simulink model "cobem_IMC"  (R2018a)
settings: Solver=FixedStepAuto  StartTime=0.0  StopTime=tfinal  FixedStep=dt  RelTol=1e-3
values from neighbouring files (symbols this model uses):
  a1 = 0.0190125110732    [PSO_workspace_PID_v1.0_agoravai_refnova.mat]    (also in cobem_IMC_script.m; teste_linearizacao.m)
  a2 = 0.594107643424    [PSO_workspace_PID_v1.0_agoravai_refnova.mat]    (also in cobem_IMC_script.m = num2/den2; teste_linearizacao.m = num2/den2)
  a3 = 0.0893725569407    [PSO_workspace_PID_v1.0_agoravai_refnova.mat]    (also in cobem_IMC_script.m = num3/den3; teste_linearizacao.m = num3/den3)
  a4 = 0.0670294177055    [PSO_workspace_PID_v1.0_agoravai_refnova.mat]    (also in cobem_IMC_script.m = num4/den4; teste_linearizacao.m = num4/den4)
  h10 = 0.3    [PSO_workspace_PID_v1.0_agoravai_refnova.mat]    (also in cobem_IMC_script.m)
  H1max = 1    [PSO_workspace_PID_v1.0_agoravai_refnova.mat]    (also in cobem_IMC_script.m; teste_linearizacao.m)
  h20 = 0.1    [PSO_workspace_PID_v1.0_agoravai_refnova.mat]    (also in cobem_IMC_script.m)
  H2max = 1    [PSO_workspace_PID_v1.0_agoravai_refnova.mat]    (also in cobem_IMC_script.m; teste_linearizacao.m)
  KpIMC = (tau1+tau2)/(K*lambda)    [cobem_IMC_script.m]
  N = 100    [PSO_workspace_PID_v1.0_agoravai_refnova.mat]    (also in cobem_IMC_script.m)
  satF_inf = 10    [PSO_workspace_PID_v1.0_agoravai_refnova.mat]    (also in cobem_IMC_script.m)
  satF_sup = 90    [PSO_workspace_PID_v1.0_agoravai_refnova.mat]    (also in cobem_IMC_script.m)
  TdIMC = (tau1*tau2)/(tau1+tau2)    (= 1.32135382724)    [cobem_IMC_script.m]
  TiIMC = (tau1+tau2)    (= 6.506)    [cobem_IMC_script.m]
settings Model: Creator=generic-user  LastModifiedBy=generic-user

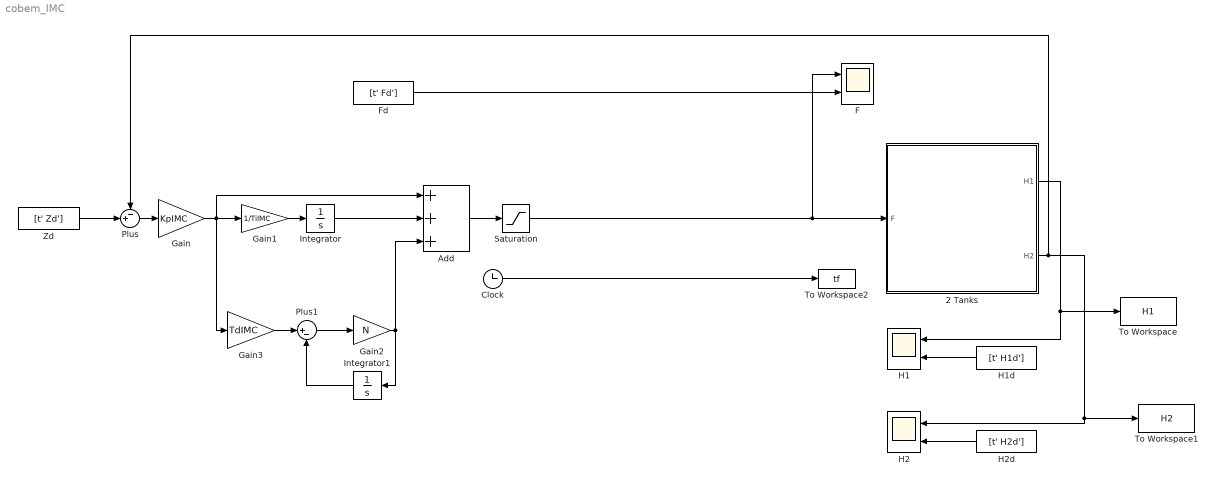
== system cobem_IMC ==
  2 Tanks : Subsystem
  Add : Sum  Inputs=3
  Clock : Clock
  F : Scope  NumInputPorts=2
  Fd : FromWorkspace  VariableName=[t' Fd']  SampleTime=0  OutputAfterFinalValue=Holding final value
  Gain : Gain  Gain=KpIMC
  Gain1 : Gain  Gain=1/TiIMC
  Gain2 : Gain  Gain=N
  Gain3 : Gain  Gain=TdIMC
  H1 : Scope  NumInputPorts=2
  H1d : FromWorkspace  VariableName=[t' H1d']  SampleTime=0  OutputAfterFinalValue=Holding final value
  H2 : Scope  NumInputPorts=2
  H2d : FromWorkspace  VariableName=[t' H2d']  SampleTime=0  OutputAfterFinalValue=Holding final value
  Integrator : Integrator
  Integrator1 : Integrator
  Plus : Sum  Inputs=-+|
  Plus1 : Sum  Inputs=|+-
  Saturation : Saturate  UpperLimit=satF_sup  LowerLimit=satF_inf
  To Workspace : ToWorkspace  VariableName=H1  SampleTime=-1
  To Workspace1 : ToWorkspace  VariableName=H2  SampleTime=-1
  To Workspace2 : ToWorkspace  VariableName=tf  SampleTime=-1
  Zd : FromWorkspace  VariableName=[t' Zd']  SampleTime=0  OutputAfterFinalValue=Holding final value
  wires:
  Zd/1 -> Plus/2
  H2d/1 -> H2/2
  2 Tanks/1(H1) -> To Workspace/1, H1/1
  Plus/1 -> Gain/1
  Fd/1 -> F/2
  Clock/1 -> To Workspace2/1
  2 Tanks/2(H2) -> To Workspace1/1, H2/1, Plus/1
  H1d/1 -> H1/2
  Add/1 -> Saturation/1
  Integrator/1 -> Add/2
  Gain/1 -> Gain3/1, Add/1, Gain1/1
  Gain1/1 -> Integrator/1
  Integrator1/1 -> Plus1/2
  Plus1/1 -> Gain2/1
  Gain2/1 -> Integrator1/1, Add/3
  Gain3/1 -> Plus1/1
  Saturation/1 -> F/1, 2 Tanks/1(F)

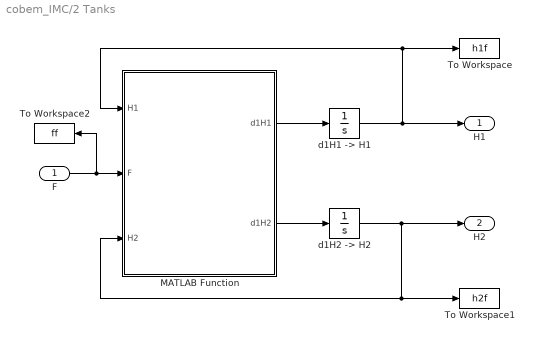
== system cobem_IMC/2 Tanks ==
  F : Inport
  MATLAB Function : MATLAB Function  TreatAsAtomicUnit=on
  To Workspace : ToWorkspace  VariableName=h1f  SampleTime=-1
  To Workspace1 : ToWorkspace  VariableName=h2f  SampleTime=-1
  To Workspace2 : ToWorkspace  VariableName=ff  SampleTime=-1
  "d1H1 -> H1" : Integrator  InitialCondition=h10  LimitOutput=on  UpperSaturationLimit=H1max  LowerSaturationLimit=0
  "d1H2 -> H2" : Integrator  InitialCondition=h20  LimitOutput=on  UpperSaturationLimit=H2max  LowerSaturationLimit=0
  H1 : Outport
  H2 : Outport  Port=2
  wires:
  MATLAB Function/1(d1H1) -> "d1H1 -> H1"/1
  "d1H1 -> H1"/1 -> H1/1, To Workspace/1, MATLAB Function/1(H1)
  MATLAB Function/2(d1H2) -> "d1H2 -> H2"/1
  F/1 -> To Workspace2/1, MATLAB Function/2(F)
  "d1H2 -> H2"/1 -> H2/1, To Workspace1/1, MATLAB Function/3(H2)

== matlab function cobem_IMC/2 Tanks/MATLAB Function ==
  data: H1 input; F input; d1H1 output; H2 input; d1H2 output; a1 parameter; a2 parameter; a3 parameter; a4 parameter
function [d1H1, d1H2] = TwoTanks(H1, F, H2, a1, a2, a3, a4)
  
  % Sistema Dinâmico
    d1H1 = a1*F - a2*sqrt(H1);
    
    d1H2 = a3*(sqrt(H1)/(H2^2)) - a4*(1/(H2^1.5));
